simulink model "AFDNFSmodelMPA"  (Simulink 8.8)
settings: Solver=ode45  StartTime=0.0  StopTime=100  FixedStep=1e-3  RelTol=1e-6  EnableMultiTasking=on
InitFcn:
  | run('Methods/AFDSimInit')
  | load('SampleDatcomData.mat')
values from neighbouring files (symbols this model uses):
  nfs = TransferFunction('Plot','true')    [Main.m]    (also in NFSDatabase.sldd = SI
                Imperial
                28184.4409185639)
undefined symbols (not defined in the file or in its folder): datcom, desired, K_lat, K_long, Kobsvlat, Kobsvlong, lat, latsys, long, longsys, Newton, Raphson, sigbuilder_block
libraries: aerolibutil x13, aerolibtransform2 x1, aerolibasang x1
(part 2 of 3)

== system AFDNFSmodelMPA/Nonlinear Flight Simulator/Forces&Moments/Aero Attributes/Velocity Magnitude ==
  Velocity : Inport
  Dot Product : DotProduct  InputSameDT=on  OutDataTypeStr=Inherit: Inherit via internal rule
  Sqrt : Sqrt  SaturateOnIntegerOverflow=on
  Velocity Magnitude : Outport
  wires:
  Sqrt/1 -> Velocity Magnitude/1  "abs(V)"
  Velocity/1 -> Dot Product/2, Dot Product/1
  Dot Product/1 -> Sqrt/1

== system AFDNFSmodelMPA/Nonlinear Flight Simulator/Forces&Moments/Digital DATCOM v1.0.2/Deflection ==
  CP : Inport
  bus : Inport  Port=2
  "V " : Inport  Port=3
  qbar : Inport  Port=4
  CG : Inport  Port=5
  S ref : Inport  Port=6  Unit=m^2
  b ref : Inport  Port=7  Unit=m  PortDimensions=1
  c bar : Inport  Port=8  Unit=m  PortDimensions=1
  Aerodynamic Forces and Moments : Subsystem
  Delta Coefficients : Subsystem
  delta_Faero : Outport
  delta_Maero : Outport  Port=2
  wires:
  Aerodynamic Forces and Moments/1(Forces) -> delta_Faero/1
  Aerodynamic Forces and Moments/2(Moments) -> delta_Maero/1
  S ref/1 -> Aerodynamic Forces and Moments/6(S ref)
  b ref/1 -> Aerodynamic Forces and Moments/7(b ref)
  qbar/1 -> Aerodynamic Forces and Moments/2(qbar)
  c bar/1 -> Aerodynamic Forces and Moments/8(cbar)
  CG/1 -> Aerodynamic Forces and Moments/3(CG)
  "V "/1 -> Aerodynamic Forces and Moments/5(Vb)
  CP/1 -> Aerodynamic Forces and Moments/4(CP)
  Delta Coefficients/1(delCoeff) -> Aerodynamic Forces and Moments/1(Coefficients)
  bus/1 -> Delta Coefficients/1(bus)

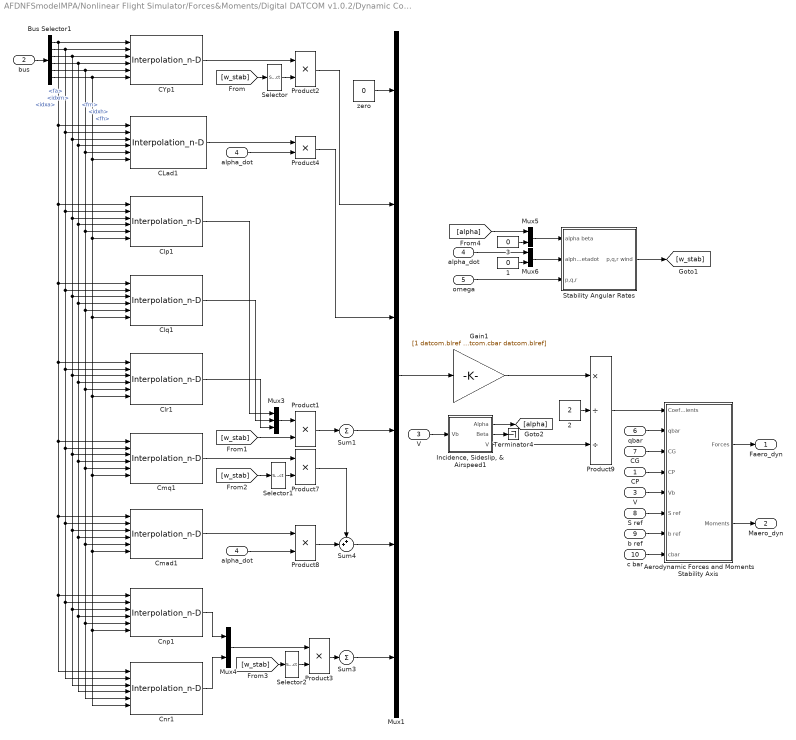
== system AFDNFSmodelMPA/Nonlinear Flight Simulator/Forces&Moments/Digital DATCOM v1.0.2/Dynamic Contribution ==
  CP : Inport
  bus : Inport  Port=2
  V : Inport  Port=3
  alpha_dot : Inport  Port=4  Unit=rad/s
  omega : Inport  Port=5  Unit=rad/s
  qbar : Inport  Port=6
  CG : Inport  Port=7
  S ref : Inport  Port=8  Unit=m^2
  b ref : Inport  Port=9  Unit=m  PortDimensions=1
  c bar : Inport  Port=10  Unit=m  PortDimensions=1
  " V " : InportShadow  Port=3
  " alpha_dot " : InportShadow  Port=4  Unit=rad/s
  1 : Constant  Value=0
  2 : Constant  Value=2
  3 : Constant  Value=0
  Aerodynamic Forces and Moments Stability Axis : Subsystem
  Bus Selector1 : BusSelector  OutputSignals=idxa,fa,idxm,fm,idxh,fh
  CLad1 : Interpolation_n-D  NumberOfTableDimensions=3  Table="permute(datcom.clad,[1  2  3])"  OutDataTypeStr=double
      settings: InputPortMap=u0,u1,u2,u3,u4,u5
  CYp1 : Interpolation_n-D  NumberOfTableDimensions=3  Table="permute(datcom.cyp,[1  2  3])"  OutDataTypeStr=double
      settings: InputPortMap=u0,u1,u2,u3,u4,u5
  Clp1 : Interpolation_n-D  NumberOfTableDimensions=3  Table="permute(datcom.clp,[1  2  3])"  OutDataTypeStr=double
      settings: InputPortMap=u0,u1,u2,u3,u4,u5
  Clq1 : Interpolation_n-D  NumberOfTableDimensions=3  Table="permute(datcom.clq,[1  2  3])"  OutDataTypeStr=double
      settings: InputPortMap=u0,u1,u2,u3,u4,u5
  Clr1 : Interpolation_n-D  NumberOfTableDimensions=3  Table="permute(datcom.clr,[1  2  3])"  OutDataTypeStr=double
      settings: InputPortMap=u0,u1,u2,u3,u4,u5
  Cmad1 : Interpolation_n-D  NumberOfTableDimensions=3  Table="permute(datcom.cmad,[1  2  3])"  OutDataTypeStr=double
      settings: InputPortMap=u0,u1,u2,u3,u4,u5
  Cmq1 : Interpolation_n-D  NumberOfTableDimensions=3  Table="permute(datcom.cmq,[1  2  3])"  OutDataTypeStr=double
      settings: InputPortMap=u0,u1,u2,u3,u4,u5
  Cnp1 : Interpolation_n-D  NumberOfTableDimensions=3  Table="permute(datcom.cnp,[1  2  3])"  OutDataTypeStr=double
      settings: InputPortMap=u0,u1,u2,u3,u4,u5
  Cnr1 : Interpolation_n-D  NumberOfTableDimensions=3  Table="permute(datcom.cnr,[1  2  3])"  OutDataTypeStr=double
      settings: InputPortMap=u0,u1,u2,u3,u4,u5
  Gain1 : Gain  Gain=[1 datcom.blref datcom.cbar datcom.blref datcom.cbar datcom.blref]
  "Incidence, Sideslip, & Airspeed1" : Subsystem
      mask Display:
      | port_label('input',1,'V_b','texmode','on');
      | port_label('output',1,'\alpha','texmode','on');
      | port_label('output',2,'\beta','texmode','on');
      | port_label('output',3,'V','texmode','on');
  Mux1 : Mux  Inputs=6
  Mux3 : Mux  Inputs=3
  Mux4 : Mux  Inputs=2
  Mux5 : Mux  Inputs=2
  Mux6 : Mux  Inputs=2
  Product{1..4,7..8} (6 alike) : Product  RndMeth=Zero
  Product9 : Product  Inputs=*//  RndMeth=Zero
  Selector : Selector  InputPortWidth=3  IndexOptions=Index vector (dialog)  Indices=1  OutputSizes=1
  Selector1 : Selector  InputPortWidth=3  IndexOptions=Index vector (dialog)  Indices=2  OutputSizes=1
  Selector2 : Selector  InputPortWidth=3  IndexOptions=Index vector (dialog)  Indices=[1 3]  OutputSizes=1
  Stability Angular Rates : Subsystem
      mask Display:
      | port_label('input',1,'\alpha \beta','texmode','on');
      | port_label('input',2,'d\alpha/dt d\beta/dt','texmode','on');
      | port_label('input',3,'\omega','texmode','on');
      | port_label('output',1,'\omega_w','texmode','on');
  Sum1 : Sum  Inputs=+
  Sum3 : Sum  Inputs=+
  Sum4 : Sum  Inputs=++|
  Terminator4 : Terminator
  "alpha_dot " : InportShadow  Port=4  Unit=rad/s
  zero : Constant  Value=0
  Faero_dyn : Outport
  Maero_dyn : Outport  Port=2
  wires:
  c bar/1 -> Aerodynamic Forces and Moments Stability Axis/8(cbar)
  b ref/1 -> Aerodynamic Forces and Moments Stability Axis/7(b ref)
  S ref/1 -> Aerodynamic Forces and Moments Stability Axis/6(S ref)
  CLad1/1 -> Product4/1
  Bus Selector1/6 -> Clp1/6, Clq1/6, Clr1/6, Cmq1/6, Cmad1/6, Cnp1/6, Cnr1/6, CLad1/6, CYp1/6  "<fh>"
  Bus Selector1/5 -> Clp1/5, Clq1/5, Clr1/5, Cmq1/5, Cmad1/5, Cnp1/5, Cnr1/5, CLad1/5, CYp1/5  "<idxh>"
  Bus Selector1/4 -> Clp1/4, Clq1/4, Clr1/4, Cmq1/4, Cmad1/4, Cnp1/4, Cnr1/4, CLad1/4, CYp1/4  "<fm>"
  Bus Selector1/3 -> Clp1/3, Clq1/3, Clr1/3, Cmq1/3, Cmad1/3, Cnp1/3, Cnr1/3, CLad1/3, CYp1/3  "<idxm>"
  Bus Selector1/2 -> Clp1/2, Clq1/2, Clr1/2, Cmq1/2, Cmad1/2, Cnp1/2, Cnr1/2, CLad1/2, CYp1/2  "<fa>"
  Bus Selector1/1 -> Clp1/1, Clq1/1, Clr1/1, Cmq1/1, Cmad1/1, Cnp1/1, Cnr1/1, CLad1/1, CYp1/1  "<idxa>"
  bus/1 -> Bus Selector1/1
  " alpha_dot "/1 -> Mux6/1
  omega/1 -> Stability Angular Rates/3(p,q,r)
  Stability Angular Rates/1(p,q,r wind) -> [w_stab]
  Mux1/1 -> Gain1/1
  Cnp1/1 -> Mux4/1
  Cmq1/1 -> Product7/1
  Sum1/1 -> Mux1/4
  Product2/1 -> Mux1/2
  Clq1/1 -> Mux3/2
  Selector/1 -> Product2/2
  CYp1/1 -> Product2/1
  "alpha_dot "/1 -> Product4/2
  [w_stab] -> Selector/1
  Clr1/1 -> Mux3/3
  Clp1/1 -> Mux3/1
  Mux3/1 -> Product1/1
  [w_stab] -> Product1/2
  Product1/1 -> Sum1/1
  [w_stab] -> Selector1/1
  Selector1/1 -> Product7/2
  Product7/1 -> Sum4/1
  Cmad1/1 -> Product8/1
  Product8/1 -> Sum4/2
  alpha_dot/1 -> Product8/2
  Cnr1/1 -> Mux4/2
  [w_stab] -> Selector2/1
  Mux4/1 -> Product3/1
  Selector2/1 -> Product3/2
  Sum3/1 -> Mux1/6
  Product3/1 -> Sum3/1
  Gain1/1 -> Product9/1
  Product9/1 -> Aerodynamic Forces and Moments Stability Axis/1(Coefficients)
  2/1 -> Product9/2
  V/1 -> "Incidence, Sideslip, & Airspeed1"/1(Vb)
  Sum4/1 -> Mux1/5
  Product4/1 -> Mux1/3
  zero/1 -> Mux1/1
  "Incidence, Sideslip, & Airspeed1"/3(V) -> Product9/3
  "Incidence, Sideslip, & Airspeed1"/2(Beta) -> Terminator4/1
  "Incidence, Sideslip, & Airspeed1"/1(Alpha) -> [alpha]
  Aerodynamic Forces and Moments Stability Axis/1(Forces) -> Faero_dyn/1
  qbar/1 -> Aerodynamic Forces and Moments Stability Axis/2(qbar)
  Aerodynamic Forces and Moments Stability Axis/2(Moments) -> Maero_dyn/1
  " V "/1 -> Aerodynamic Forces and Moments Stability Axis/5(Vb)
  3/1 -> Mux5/2
  [alpha] -> Mux5/1
  Mux5/1 -> Stability Angular Rates/1(alpha beta)
  Mux6/1 -> Stability Angular Rates/2(alphadot betadot)
  1/1 -> Mux6/2
  CG/1 -> Aerodynamic Forces and Moments Stability Axis/3(CG)
  CP/1 -> Aerodynamic Forces and Moments Stability Axis/4(CP)

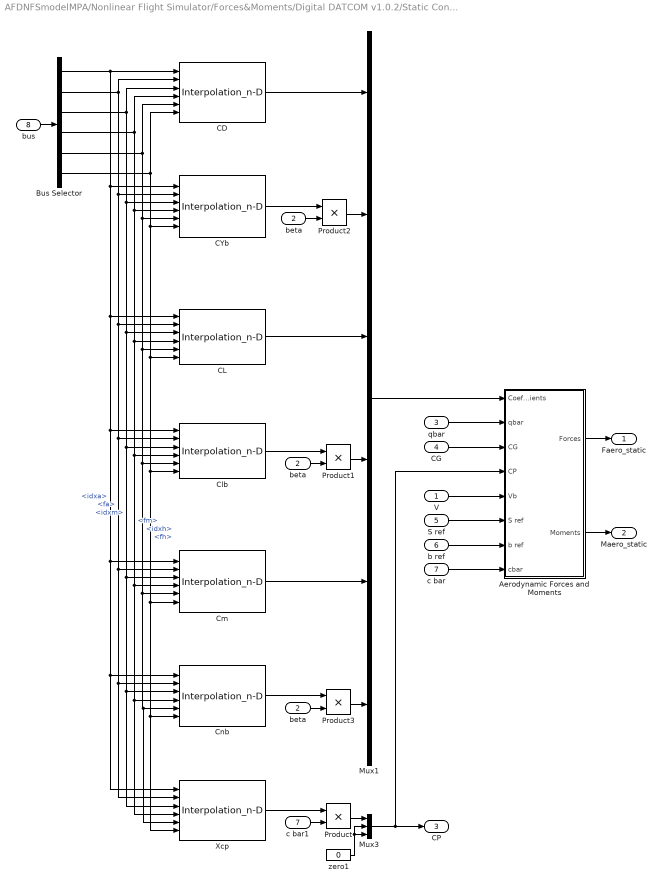
== system AFDNFSmodelMPA/Nonlinear Flight Simulator/Forces&Moments/Digital DATCOM v1.0.2/Static Contribution ==
  "V " : Inport
  beta : Inport  Port=2
  qbar : Inport  Port=3
  CG : Inport  Port=4
  S ref : Inport  Port=5  Unit=m^2
  b ref : Inport  Port=6  Unit=m  PortDimensions=1
  c bar : Inport  Port=7  Unit=m  PortDimensions=1
  bus : Inport  Port=8
  " beta " : InportShadow  Port=2
  Aerodynamic Forces and Moments : Subsystem
  Bus Selector : BusSelector  OutputSignals=idxa,fa,idxm,fm,idxh,fh
  CD : Interpolation_n-D  NumberOfTableDimensions=3  Table=permute(datcom.cd,[1 2 3])  InterpMethod=Flat  ExtrapMethod=Clip  OutDataTypeStr=double
      settings: InputPortMap=u0,u1,u2,u3,u4,u5
  CL : Interpolation_n-D  NumberOfTableDimensions=3  Table=permute(datcom.cl,[1 2 3])  InterpMethod=Flat  ExtrapMethod=Clip  OutDataTypeStr=double
      settings: InputPortMap=u0,u1,u2,u3,u4,u5
  CYb : Interpolation_n-D  NumberOfTableDimensions=3  Table=permute(datcom.cyb,[1 2 3])  InterpMethod=Flat  ExtrapMethod=Clip  OutDataTypeStr=double
      settings: InputPortMap=u0,u1,u2,u3,u4,u5
  Clb : Interpolation_n-D  NumberOfTableDimensions=3  Table=permute(datcom.clb,[1 2 3])  InterpMethod=Flat  ExtrapMethod=Clip  OutDataTypeStr=double
      settings: InputPortMap=u0,u1,u2,u3,u4,u5
  Cm : Interpolation_n-D  NumberOfTableDimensions=3  Table=permute(datcom.cm,[1 2 3])  InterpMethod=Flat  ExtrapMethod=Clip  OutDataTypeStr=double
      settings: InputPortMap=u0,u1,u2,u3,u4,u5
  Cnb : Interpolation_n-D  NumberOfTableDimensions=3  Table=permute(datcom.cnb,[1 2 3])  InterpMethod=Flat  ExtrapMethod=Clip  OutDataTypeStr=double
      settings: InputPortMap=u0,u1,u2,u3,u4,u5
  Mux1 : Mux  Inputs=6
  Mux3 : Mux  Inputs=3
  Product : Product
  Product1 : Product  RndMeth=Zero
  Product2 : Product  RndMeth=Zero
  Product3 : Product  RndMeth=Zero
  Xcp : Interpolation_n-D  NumberOfTableDimensions=3  Table="permute(datcom.xcp,[1  2  3])"  OutDataTypeStr=double
      settings: InputPortMap=u0,u1,u2,u3,u4,u5
  "beta " : InportShadow  Port=2
  c bar1 : InportShadow  Port=7  Unit=m  PortDimensions=1
  zero1 : Constant  Value=0
  Faero_static : Outport
  Maero_static : Outport  Port=2
  "CP " : Outport  Port=3
  wires:
  c bar1/1 -> Product/2
  Product/1 -> Mux3/1
  zero1/1 -> Mux3/3, Mux3/2
  Xcp/1 -> Product/1
  c bar/1 -> Aerodynamic Forces and Moments/8(cbar)
  b ref/1 -> Aerodynamic Forces and Moments/7(b ref)
  S ref/1 -> Aerodynamic Forces and Moments/6(S ref)
  Mux3/1 -> Aerodynamic Forces and Moments/4(CP), "CP "/1
  CG/1 -> Aerodynamic Forces and Moments/3(CG)
  bus/1 -> Bus Selector/1
  Bus Selector/1 -> CD/1, CYb/1, Clb/1, Cnb/1, Xcp/1, Cm/1, CL/1  "<idxa>"
  Bus Selector/2 -> Cnb/2, Xcp/2, Cm/2, Clb/2, CL/2, CYb/2, CD/2  "<fa>"
  Bus Selector/3 -> Cnb/3, Xcp/3, Cm/3, Clb/3, CL/3, CYb/3, CD/3  "<idxm>"
  Bus Selector/4 -> Cnb/4, Xcp/4, Cm/4, Clb/4, CL/4, CYb/4, CD/4  "<fm>"
  Bus Selector/5 -> Cnb/5, Xcp/5, Cm/5, Clb/5, CL/5, CYb/5, CD/5  "<idxh>"
  Bus Selector/6 -> Cnb/6, Xcp/6, Cm/6, Clb/6, CL/6, CYb/6, CD/6  "<fh>"
  CD/1 -> Mux1/1
  CL/1 -> Mux1/3
  CYb/1 -> Product2/1
  beta/1 -> Product2/2
  Clb/1 -> Product1/1
  "beta "/1 -> Product1/2
  Product2/1 -> Mux1/2
  Product1/1 -> Mux1/4
  Cm/1 -> Mux1/5
  Cnb/1 -> Product3/1
  " beta "/1 -> Product3/2
  Product3/1 -> Mux1/6
  Mux1/1 -> Aerodynamic Forces and Moments/1(Coefficients)
  Aerodynamic Forces and Moments/1(Forces) -> Faero_static/1
  qbar/1 -> Aerodynamic Forces and Moments/2(qbar)
  Aerodynamic Forces and Moments/2(Moments) -> Maero_static/1
  "V "/1 -> Aerodynamic Forces and Moments/5(Vb)

== system AFDNFSmodelMPA/Nonlinear Flight Simulator/Forces&Moments/Thrust/Signal Builder ==
  Demux : Demux  Tag=STV Demux  Outputs=1
  FromWs : FromWorkspace  Tag=STV FromWs  VariableName=tuvar  SampleTime=0  SigBuilderData=DataTag1  VnvData=DataTag2
      SigBuilderData=|
      | common.afterFinalStr = 'Extrapolate'
      | common.sampleTime = 0
      | dataSet.timeRange = [0 1200]
      | dataSet.name = 'Thrust Deviation'
      | sbobj.Groups.Name = 'Thrust Deviation'
      | sbobj.Groups.Signals.Name = 'ThrustDeviation'
      | sbobj.Groups.Signals.XData = [0 10 10 12 12 1200]
      | sbobj.Groups.Signals.YData = [1 1 1.05 1.05 1 1]
      | sbobj.Groups.TimeRange = [0 1200]
  ThrustDeviation : Outport  Tag=STV Outport
  wires:
  Demux/1 -> ThrustDeviation/1
  FromWs/1 -> Demux/1

== system AFDNFSmodelMPA/OnBoardComputer/Control System/Trim/Doublet Generated Signal ==
  Constant : Constant  Value=[0;0;0]
  Constant2 : Constant  Value=nfs.trim.delta_e
  Doublet : Subsystem  mask{T_start=10, amp=deg2rad(2), span=1, sampletime=0}
      mask prompts: T_start "Doublet Time"; amp "Amplitude"; span "Time Span"; sampletime "Sample Time"
      mask Display: plot([0,1,1,2,2,3,3,4],[0,0,1,1,-1,-1,0,0])
  Mux : Mux  Inputs=2
  Sum : Sum  Inputs=|++
  Doublet Out : Outport
  wires:
  Sum/1 -> Mux/1
  Constant/1 -> Mux/2
  Doublet/1(Out1) -> Sum/1
  Constant2/1 -> Sum/2
  Mux/1 -> Doublet Out/1

== system AFDNFSmodelMPA/OnBoardComputer/Control System/Trim/Triangular signal span 10 sec ==
  Bus Creator : BusCreator  Inputs=4
  Constant1 : Constant  Value=0
  Constant2 : Constant  Value=nfs.trim.delta_e
  Constant3 : Constant  Value=0
  Constant4 : Constant  Value=0
  Gain{,1..3} (4 alike) : Gain  Gain=pi/180
  Gain4 : Gain  Gain=0
  Gain5 : Gain  Gain=0
  Gain6 : Gain  Gain=0
  Gain7 : Gain
  Signal Builder1 : Subsystem  Tag=STV Subsys  LoadFcn=sigbuilder_block('load');  StartFcn=sigbuilder_block('start');  StopFcn=sigbuilder_block('stop');  ClipboardFcn=sigbuilder_block('clipboard');  mask(Sigbuilder block){tuvar=[0:10]}
      mask help: Simulink:masks:SigbuilderBlock_MD
      mask init:
      | if ~strcmp(get_param(bdroot(gcbh),'SimulationStatus'),'stopped') tuvar = sigbuilder_block('maskInit'); end
      settings: CopyFcn=sigbuilder_block('copy');  DeleteFcn=sigbuilder_block('delete');  ModelCloseFcn=sigbuilder_block('modelClose');  PreSaveFcn=sigbuilder_block('preSave');  PauseFcn=sigbuilder_block('pause');  ContinueFcn=sigbuilder_block('continue');  NameChangeFcn=sigbuilder_block('namechange');  OpenFcn=sigbuilder_block('open',[437.4 199.2 550.2 400.2 ]);  CloseFcn=sigbuilder_block('close');
      mask Display: plot(0, 0, 100, 100,[2, 2, 32, 32, 2], [68, 8, 8, 68, 68],[32, 2], [38, 38], [32, 19, 2],[53, 60, 44], [32, 17, 17, 2],[16, 16, 31, 31]);txt = getActiveGroup(gcbh);text(2, 100, txt,'verticalAlignment', 'top');
  Signal Builder2 : Subsystem  Tag=STV Subsys  LoadFcn=sigbuilder_block('load');  StartFcn=sigbuilder_block('start');  StopFcn=sigbuilder_block('stop');  ClipboardFcn=sigbuilder_block('clipboard');  mask(Sigbuilder block){tuvar=[0:10]}
      mask help: Simulink:masks:SigbuilderBlock_MD
      mask init:
      | if ~strcmp(get_param(bdroot(gcbh),'SimulationStatus'),'stopped') tuvar = sigbuilder_block('maskInit'); end
      settings: CopyFcn=sigbuilder_block('copy');  DeleteFcn=sigbuilder_block('delete');  ModelCloseFcn=sigbuilder_block('modelClose');  PreSaveFcn=sigbuilder_block('preSave');  PauseFcn=sigbuilder_block('pause');  ContinueFcn=sigbuilder_block('continue');  NameChangeFcn=sigbuilder_block('namechange');  OpenFcn=sigbuilder_block('open',[437.25 199.5 550.5 399.75 ]);  CloseFcn=sigbuilder_block('close');
      mask Display: plot(0, 0, 100, 100,[2, 2, 32, 32, 2], [68, 8, 8, 68, 68],[32, 2], [38, 38], [32, 19, 2],[53, 60, 44], [32, 17, 17, 2],[16, 16, 31, 31]);txt = getActiveGroup(gcbh);text(2, 100, txt,'verticalAlignment', 'top');
  Signal Builder3 : Subsystem  Tag=STV Subsys  LoadFcn=sigbuilder_block('load');  StartFcn=sigbuilder_block('start');  StopFcn=sigbuilder_block('stop');  ClipboardFcn=sigbuilder_block('clipboard');  mask(Sigbuilder block){tuvar=[0:10]}
      mask help: Simulink:masks:SigbuilderBlock_MD
      mask init:
      | if ~strcmp(get_param(bdroot(gcbh),'SimulationStatus'),'stopped') tuvar = sigbuilder_block('maskInit'); end
      settings: CopyFcn=sigbuilder_block('copy');  DeleteFcn=sigbuilder_block('delete');  ModelCloseFcn=sigbuilder_block('modelClose');  PreSaveFcn=sigbuilder_block('preSave');  PauseFcn=sigbuilder_block('pause');  ContinueFcn=sigbuilder_block('continue');  NameChangeFcn=sigbuilder_block('namechange');  OpenFcn=sigbuilder_block('open',[437.25 199.5 550.5 399.75 ]);  CloseFcn=sigbuilder_block('close');
      mask Display: plot(0, 0, 100, 100,[2, 2, 32, 32, 2], [68, 8, 8, 68, 68],[32, 2], [38, 38], [32, 19, 2],[53, 60, 44], [32, 17, 17, 2],[16, 16, 31, 31]);txt = getActiveGroup(gcbh);text(2, 100, txt,'verticalAlignment', 'top');
  Signal Builder4 : Subsystem  Tag=STV Subsys  LoadFcn=sigbuilder_block('load');  StartFcn=sigbuilder_block('start');  StopFcn=sigbuilder_block('stop');  ClipboardFcn=sigbuilder_block('clipboard');  mask(Sigbuilder block){tuvar=[0:10]}
      mask help: Simulink:masks:SigbuilderBlock_MD
      mask init:
      | if ~strcmp(get_param(bdroot(gcbh),'SimulationStatus'),'stopped') tuvar = sigbuilder_block('maskInit'); end
      settings: CopyFcn=sigbuilder_block('copy');  DeleteFcn=sigbuilder_block('delete');  ModelCloseFcn=sigbuilder_block('modelClose');  PreSaveFcn=sigbuilder_block('preSave');  PauseFcn=sigbuilder_block('pause');  ContinueFcn=sigbuilder_block('continue');  NameChangeFcn=sigbuilder_block('namechange');  OpenFcn=sigbuilder_block('open',[437.25 199.5 550.5 399.75 ]);  CloseFcn=sigbuilder_block('close');
      mask Display: plot(0, 0, 100, 100,[2, 2, 32, 32, 2], [68, 8, 8, 68, 68],[32, 2], [38, 38], [32, 19, 2],[53, 60, 44], [32, 17, 17, 2],[16, 16, 31, 31]);txt = getActiveGroup(gcbh);text(2, 100, txt,'verticalAlignment', 'top');
  Sum{,1..3} (4 alike) : Sum  Inputs=++|
  Tri : Outport
  wires:
  Signal Builder1/1(Normalized Elevator(deg)) -> Gain/1
  Constant2/1 -> Sum/1
  Gain/1 -> Sum/2
  Signal Builder2/1(Normalized Flap(deg)) -> Gain1/1
  Constant1/1 -> Sum1/1
  Gain1/1 -> Sum1/2
  Signal Builder3/1(Normalized Alileron(deg)) -> Gain2/1
  Constant3/1 -> Sum2/1
  Gain2/1 -> Sum2/2
  Signal Builder4/1(Normalized Rudder(deg)) -> Gain3/1
  Constant4/1 -> Sum3/1
  Gain3/1 -> Sum3/2
  Sum/1 -> Gain7/1
  Sum1/1 -> Gain6/1
  Sum2/1 -> Gain5/1
  Sum3/1 -> Gain4/1
  Gain6/1 -> Bus Creator/2  "delta_f"
  Gain5/1 -> Bus Creator/3  "delta_a"
  Gain7/1 -> Bus Creator/1  "delta_e"
  Gain4/1 -> Bus Creator/4  "delta_r"
  Bus Creator/1 -> Tri/1

== system AFDNFSmodelMPA/Nonlinear Flight Simulator/6DoF Nonlinear Flight Equations of Motion (Rigid Body)/AngularAcceleration(Omegadot)/Cross Product/Subsystem2 ==
  A : Inport
  B : Inport  Port=2
  Demux : Demux  Outputs=3
  Demux1 : Demux  Outputs=3
  Mux : Mux  Inputs=3
  i x j : Product  SaturateOnIntegerOverflow=on  InputSameDT=on  OutDataTypeStr=Inherit: Same as first input
  j x k : Product  SaturateOnIntegerOverflow=on  InputSameDT=on  OutDataTypeStr=Inherit: Same as first input
  k x i : Product  SaturateOnIntegerOverflow=on  InputSameDT=on  OutDataTypeStr=Inherit: Same as first input
  Out1 : Outport
  wires:
  Demux1/3 -> j x k/2
  Demux/2 -> j x k/1
  Demux/3 -> k x i/1
  Demux1/1 -> k x i/2
  Demux1/2 -> i x j/2
  Demux/1 -> i x j/1
  i x j/1 -> Mux/3
  k x i/1 -> Mux/2
  j x k/1 -> Mux/1
  B/1 -> Demux1/1
  A/1 -> Demux/1
  Mux/1 -> Out1/1

== system AFDNFSmodelMPA/Nonlinear Flight Simulator/6DoF Nonlinear Flight Equations of Motion (Rigid Body)/AngularAcceleration(Omegadot)/Cross Product/Subsystem3 ==
  A : Inport
  B : Inport  Port=2
  Demux : Demux  Outputs=3
  Demux1 : Demux  Outputs=3
  Mux : Mux  Inputs=3
  i x k : Product  SaturateOnIntegerOverflow=on  InputSameDT=on  OutDataTypeStr=Inherit: Same as first input
  j x i : Product  SaturateOnIntegerOverflow=on  InputSameDT=on  OutDataTypeStr=Inherit: Same as first input
  k x j : Product  SaturateOnIntegerOverflow=on  InputSameDT=on  OutDataTypeStr=Inherit: Same as first input
  Out2 : Outport
  wires:
  j x i/1 -> Mux/3
  i x k/1 -> Mux/2
  k x j/1 -> Mux/1
  Mux/1 -> Out2/1
  Demux1/1 -> j x i/2
  Demux/2 -> j x i/1
  Demux1/3 -> i x k/2
  Demux/1 -> i x k/1
  Demux1/2 -> k x j/2
  Demux/3 -> k x j/1
  B/1 -> Demux1/1
  A/1 -> Demux/1

== system AFDNFSmodelMPA/Nonlinear Flight Simulator/6DoF Nonlinear Flight Equations of Motion (Rigid Body)/Linear Acceleration(Vdot)/Cross Product/Subsystem2 ==
  A : Inport
  B : Inport  Port=2
  Demux : Demux  Outputs=3
  Demux1 : Demux  Outputs=3
  Mux : Mux  Inputs=3
  i x j : Product  SaturateOnIntegerOverflow=on  InputSameDT=on  OutDataTypeStr=Inherit: Same as first input
  j x k : Product  SaturateOnIntegerOverflow=on  InputSameDT=on  OutDataTypeStr=Inherit: Same as first input
  k x i : Product  SaturateOnIntegerOverflow=on  InputSameDT=on  OutDataTypeStr=Inherit: Same as first input
  Out1 : Outport
  wires:
  Demux1/3 -> j x k/2
  Demux/2 -> j x k/1
  Demux/3 -> k x i/1
  Demux1/1 -> k x i/2
  Demux1/2 -> i x j/2
  Demux/1 -> i x j/1
  i x j/1 -> Mux/3
  k x i/1 -> Mux/2
  j x k/1 -> Mux/1
  B/1 -> Demux1/1
  A/1 -> Demux/1
  Mux/1 -> Out1/1

== system AFDNFSmodelMPA/Nonlinear Flight Simulator/6DoF Nonlinear Flight Equations of Motion (Rigid Body)/Linear Acceleration(Vdot)/Cross Product/Subsystem3 ==
  A : Inport
  B : Inport  Port=2
  Demux : Demux  Outputs=3
  Demux1 : Demux  Outputs=3
  Mux : Mux  Inputs=3
  i x k : Product  SaturateOnIntegerOverflow=on  InputSameDT=on  OutDataTypeStr=Inherit: Same as first input
  j x i : Product  SaturateOnIntegerOverflow=on  InputSameDT=on  OutDataTypeStr=Inherit: Same as first input
  k x j : Product  SaturateOnIntegerOverflow=on  InputSameDT=on  OutDataTypeStr=Inherit: Same as first input
  Out2 : Outport
  wires:
  j x i/1 -> Mux/3
  i x k/1 -> Mux/2
  k x j/1 -> Mux/1
  Mux/1 -> Out2/1
  Demux1/1 -> j x i/2
  Demux/2 -> j x i/1
  Demux1/3 -> i x k/2
  Demux/1 -> i x k/1
  Demux1/2 -> k x j/2
  Demux/3 -> k x j/1
  B/1 -> Demux1/1
  A/1 -> Demux/1

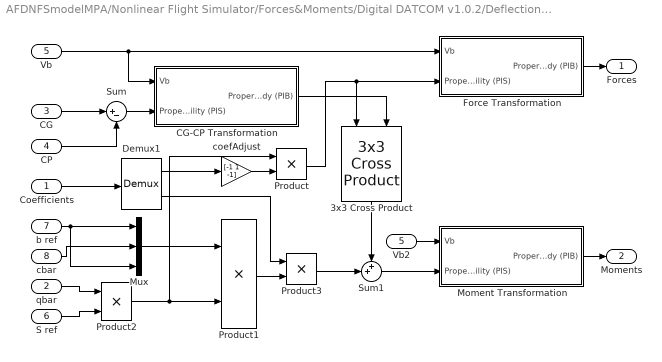
== system AFDNFSmodelMPA/Nonlinear Flight Simulator/Forces&Moments/Digital DATCOM v1.0.2/Deflection/Aerodynamic Forces and Moments ==
  Coefficients : Inport
  qbar : Inport  Port=2  Unit=Pa
  CG : Inport  Port=3  Unit=m  PortDimensions=[3, 1]
  CP : Inport  Port=4  Unit=m  PortDimensions=[3,1]
  Vb : Inport  Port=5
  S ref : Inport  Port=6  Unit=m^2  PortDimensions=1
  b ref : Inport  Port=7  Unit=m  PortDimensions=1
  cbar : Inport  Port=8  Unit=m  PortDimensions=1
  3x3 Cross Product : aerolibutil/3x3 Cross Product
  CG-CP Transformation : Subsystem
  Demux1 : Demux  Outputs=[3,3]
  Force Transformation : Subsystem
  Moment Transformation : Subsystem
  Mux : Mux  Inputs=3
  Product{,1..3} (4 alike) : Product  SaturateOnIntegerOverflow=on  InputSameDT=on  OutDataTypeStr=Inherit: Same as first input
  Sum : Sum  Inputs=|+-  SaturateOnIntegerOverflow=on
  Sum1 : Sum  Inputs=++|  SaturateOnIntegerOverflow=on  InputSameDT=on  OutDataTypeStr=Inherit: Same as first input
  Vb2 : InportShadow  Port=5
  coefAdjust : Gain  Gain="[-1  1 -1]"
  Forces : Outport  Unit=N
  Moments : Outport  Port=2  Unit=N
  wires:
  Vb2/1 -> Moment Transformation/1(Vb)
  Sum1/1 -> Moment Transformation/2(Property-In-Stability (PIS))
  S ref/1 -> Product2/2
  Mux/1 -> Product1/1
  b ref/1 -> Mux/3, Mux/1
  cbar/1 -> Mux/2
  3x3 Cross Product/1 -> Sum1/1
  Product1/1 -> Product3/2
  Coefficients/1 -> Demux1/1
  Demux1/2 -> Product3/1
  qbar/1 -> Product2/1
  Product2/1 -> Product1/2, Product/1
  Product3/1 -> Sum1/2
  Demux1/1 -> coefAdjust/1
  Product/1 -> Force Transformation/2(Property-In-Stability (PIS)), 3x3 Cross Product/1
  Force Transformation/1(Property-In-Body (PIB)) -> Forces/1
  Moment Transformation/1(Property-In-Body (PIB)) -> Moments/1
  coefAdjust/1 -> Product/2
  CG/1 -> Sum/1
  CP/1 -> Sum/2
  Sum/1 -> CG-CP Transformation/2(Property-In-Stability (PIS))
  CG-CP Transformation/1(Property-In-Body (PIB)) -> 3x3 Cross Product/2
  Vb/1 -> Force Transformation/1(Vb), CG-CP Transformation/1(Vb)

== system AFDNFSmodelMPA/Nonlinear Flight Simulator/Forces&Moments/Digital DATCOM v1.0.2/Deflection/Delta Coefficients ==
  bus : Inport
  Aileron Deflaction : Subsystem
  Elevator Deflaction : Subsystem
  Flap Deflaction : Subsystem
  Sum : Sum  Inputs=+++
  delCoeff : Outport
  wires:
  Sum/1 -> delCoeff/1
  Aileron Deflaction/1(delCoeff_a) -> Sum/3
  Flap Deflaction/1(delCoeff_f) -> Sum/1
  Elevator Deflaction/1(delCoeff_e) -> Sum/2
  bus/1 -> Elevator Deflaction/1(bus), Aileron Deflaction/1(bus), Flap Deflaction/1(bus)

== system AFDNFSmodelMPA/Nonlinear Flight Simulator/Forces&Moments/Digital DATCOM v1.0.2/Dynamic Contribution/Aerodynamic Forces and Moments Stability Axis ==
  Coefficients : Inport
  qbar : Inport  Port=2  Unit=Pa
  CG : Inport  Port=3  Unit=m  PortDimensions=[3, 1]
  CP : Inport  Port=4  Unit=m  PortDimensions=[3,1]
  Vb : Inport  Port=5
  S ref : Inport  Port=6  Unit=m^2  PortDimensions=1
  b ref : Inport  Port=7  Unit=m  PortDimensions=1
  cbar : Inport  Port=8  Unit=m  PortDimensions=1
  3x3 Cross Product : aerolibutil/3x3 Cross Product
  CG-CP Transformation : Subsystem
  Demux1 : Demux  Outputs=[3,3]
  Force Transformation : Subsystem
  Moment Transformation : Subsystem
  Mux : Mux  Inputs=3
  Product{,1..3} (4 alike) : Product  SaturateOnIntegerOverflow=on  InputSameDT=on  OutDataTypeStr=Inherit: Same as first input
  Sum : Sum  Inputs=|+-  SaturateOnIntegerOverflow=on
  Sum1 : Sum  Inputs=++|  SaturateOnIntegerOverflow=on  InputSameDT=on  OutDataTypeStr=Inherit: Same as first input
  Vb2 : InportShadow  Port=5
  coefAdjust : Gain  Gain="[-1  1 -1]"
  Forces : Outport  Unit=N
  Moments : Outport  Port=2  Unit=N*m
  wires:
  Vb2/1 -> Moment Transformation/1(Vb)
  Sum1/1 -> Moment Transformation/2(Property-In-Stability (PIS))
  S ref/1 -> Product2/2
  Mux/1 -> Product1/1
  b ref/1 -> Mux/3, Mux/1
  cbar/1 -> Mux/2
  3x3 Cross Product/1 -> Sum1/1
  Product1/1 -> Product3/2
  Coefficients/1 -> Demux1/1
  Demux1/2 -> Product3/1
  qbar/1 -> Product2/1
  Product2/1 -> Product1/2, Product/1
  Product3/1 -> Sum1/2
  Demux1/1 -> coefAdjust/1
  Product/1 -> Force Transformation/2(Property-In-Stability (PIS)), 3x3 Cross Product/1
  Force Transformation/1(Property-In-Body (PIB)) -> Forces/1
  Moment Transformation/1(Property-In-Body (PIB)) -> Moments/1
  coefAdjust/1 -> Product/2
  CG/1 -> Sum/1
  CP/1 -> Sum/2
  Sum/1 -> CG-CP Transformation/2(Property-In-Stability (PIS))
  CG-CP Transformation/1(Property-In-Body (PIB)) -> 3x3 Cross Product/2
  Vb/1 -> Force Transformation/1(Vb), CG-CP Transformation/1(Vb)

== system AFDNFSmodelMPA/Nonlinear Flight Simulator/Forces&Moments/Digital DATCOM v1.0.2/Dynamic Contribution/Incidence, Sideslip, & Airspeed1 ==
  Vb : Inport  Unit=m/s
  Airspeed : Sqrt  AlgorithmType=Newton-Raphson  SaturateOnIntegerOverflow=on
  Dot Product : DotProduct  InputSameDT=on  OutDataTypeStr=Inherit: Inherit via internal rule
  Incidence : Trigonometry  Operator=atan2
  Product : Product  Inputs=*/  SaturateOnIntegerOverflow=on  OutDataTypeStr=Inherit: Same as first input
  Selector : Selector  InputPortWidth=3  IndexOptions=Index vector (dialog)  Indices=[2]  OutputSizes=1
  Selector1 : Selector  InputPortWidth=3  IndexOptions=Index vector (dialog)  Indices=[3]  OutputSizes=1
  Selector2 : Selector  InputPortWidth=3  IndexOptions=Index vector (dialog)  Indices=[1]  OutputSizes=1
  Sideslip : Trigonometry  Operator=asin
  Alpha : Outport  Unit=rad  InitialOutput=0
  Beta : Outport  Port=2  Unit=rad  InitialOutput=0
  V : Outport  Port=3  Unit=m/s  InitialOutput=0
  wires:
  Selector/1 -> Product/1
  Sideslip/1 -> Beta/1
  Vb/1 -> Dot Product/2, Dot Product/1, Selector/1, Selector2/1, Selector1/1
  Incidence/1 -> Alpha/1
  Airspeed/1 -> V/1, Product/2
  Dot Product/1 -> Airspeed/1
  Selector2/1 -> Incidence/2
  Selector1/1 -> Incidence/1
  Product/1 -> Sideslip/1

== system AFDNFSmodelMPA/Nonlinear Flight Simulator/Forces&Moments/Digital DATCOM v1.0.2/Dynamic Contribution/Stability Angular Rates ==
  alpha beta : Inport  Unit=rad
  alphadot betadot : Inport  Port=2  Unit=rad/s
  p,q,r : Inport  Port=3  Unit=rad/s
  Demux : Demux  Outputs=2
  Direction Cosine Matrix Body to Wind : aerolibtransform2/Direction Cosine Matrix Body to Wind
  Disallow CGS : UnitConfiguration  UnitSystems=DataTag0  UnitSystemsStr=English,SI,SI (extended)  AllowAllUnitSystems=off
  Mux : Mux  Inputs=3
  Product : Product  RndMeth=Zero
  Product1 : Product  Multiplication=Matrix(*)  SaturateOnIntegerOverflow=on  InputSameDT=on  OutDataTypeStr=Inherit: Same as first input
  Product2 : Product  RndMeth=Zero
  SinCos : Trigonometry  Operator=sincos
  Subsystem : aerolibasang/Wind Angular Rates/Subsystem
  Sum : Sum  Inputs=|++
  Unary Minus : UnaryMinus
  Unary Minus1 : UnaryMinus
  p,q,r wind : Outport  Unit=rad/s  InitialOutput=0
  wires:
  alpha beta/1 -> Direction Cosine Matrix Body to Wind/1, Subsystem/1
  Subsystem/1 -> SinCos/1
  SinCos/1 -> Product/2
  SinCos/2 -> Product2/2
  Direction Cosine Matrix Body to Wind/1 -> Product1/1
  Sum/1 -> Product1/2
  Product1/1 -> p,q,r wind/1
  Mux/1 -> Sum/1
  p,q,r/1 -> Sum/2
  alphadot betadot/1 -> Demux/1
  Demux/2 -> Product2/1, Product/1
  Demux/1 -> Unary Minus/1
  Product/1 -> Unary Minus1/1
  Product2/1 -> Mux/3
  Unary Minus1/1 -> Mux/1
  Unary Minus/1 -> Mux/2

== system AFDNFSmodelMPA/Nonlinear Flight Simulator/Forces&Moments/Digital DATCOM v1.0.2/Static Contribution/Aerodynamic Forces and Moments ==
  Coefficients : Inport
  qbar : Inport  Port=2  Unit=Pa
  CG : Inport  Port=3  Unit=m  PortDimensions=[3, 1]
  CP : Inport  Port=4  Unit=m  PortDimensions=[3,1]
  Vb : Inport  Port=5
  S ref : Inport  Port=6  Unit=m^2  PortDimensions=1
  b ref : Inport  Port=7  Unit=m  PortDimensions=1
  cbar : Inport  Port=8  Unit=m  PortDimensions=1
  3x3 Cross Product : aerolibutil/3x3 Cross Product
  CG-CP Transformation : Subsystem
  Demux1 : Demux  Outputs=[3,3]
  Force Transformation : Subsystem
  Moment Transformation : Subsystem
  Mux : Mux  Inputs=3
  Product{,1..3} (4 alike) : Product  SaturateOnIntegerOverflow=on  InputSameDT=on  OutDataTypeStr=Inherit: Same as first input
  Sum : Sum  Inputs=|+-  SaturateOnIntegerOverflow=on
  Sum1 : Sum  Inputs=++|  SaturateOnIntegerOverflow=on  InputSameDT=on  OutDataTypeStr=Inherit: Same as first input
  Vb2 : InportShadow  Port=5
  coefAdjust : Gain  Gain="[-1  1 -1]"
  Forces : Outport  Unit=N
  Moments : Outport  Port=2  Unit=N*m
  wires:
  Vb2/1 -> Moment Transformation/1(Vb)
  Sum1/1 -> Moment Transformation/2(Property-In-Stability (PIS))
  S ref/1 -> Product2/2
  Mux/1 -> Product1/1
  b ref/1 -> Mux/3, Mux/1
  cbar/1 -> Mux/2
  3x3 Cross Product/1 -> Sum1/1
  Product1/1 -> Product3/2
  Coefficients/1 -> Demux1/1
  Demux1/2 -> Product3/1
  qbar/1 -> Product2/1
  Product2/1 -> Product1/2, Product/1
  Product3/1 -> Sum1/2
  Demux1/1 -> coefAdjust/1
  Product/1 -> Force Transformation/2(Property-In-Stability (PIS)), 3x3 Cross Product/1
  Force Transformation/1(Property-In-Body (PIB)) -> Forces/1
  Moment Transformation/1(Property-In-Body (PIB)) -> Moments/1
  coefAdjust/1 -> Product/2
  CG/1 -> Sum/1
  CP/1 -> Sum/2
  Sum/1 -> CG-CP Transformation/2(Property-In-Stability (PIS))
  CG-CP Transformation/1(Property-In-Body (PIB)) -> 3x3 Cross Product/2
  Vb/1 -> Force Transformation/1(Vb), CG-CP Transformation/1(Vb)

== system AFDNFSmodelMPA/OnBoardComputer/Control System/Trim/Doublet Generated Signal/Doublet ==
  Step : Step  Time=T_start  After=amp  SampleTime=sampletime
  Step1 : Step  Time=T_start+span/2  After=amp  SampleTime=sampletime
  Step2 : Step  Time=T_start+span/2  After=-amp  SampleTime=sampletime
  Step3 : Step  Time=T_start+span  After=-amp  SampleTime=sampletime
  Sum : Sum  Inputs=|+-
  Sum1 : Sum  Inputs=|+-
  Sum2 : Sum  Inputs=|++
  Out1 : Outport
  wires:
  Step/1 -> Sum/1
  Step1/1 -> Sum/2
  Step2/1 -> Sum1/1
  Step3/1 -> Sum1/2
  Sum/1 -> Sum2/1
  Sum1/1 -> Sum2/2
  Sum2/1 -> Out1/1

== system AFDNFSmodelMPA/OnBoardComputer/Control System/Trim/Triangular signal span 10 sec/Signal Builder1 ==
  Demux : Demux  Tag=STV Demux  Outputs=1
  FromWs : FromWorkspace  Tag=STV FromWs  VariableName=tuvar  SampleTime=0  SigBuilderData=DataTag3  VnvData=DataTag4
      SigBuilderData=|
      | common.afterFinalStr = 'Extrapolate'
      | common.sampleTime = 0
      | dataSet.timeRange = [10 20]
      | dataSet.name = 'Group 1'
      | sbobj.Groups.Name = 'Group 1'
      | sbobj.Groups.Signals.Name = 'Normalized Elevator(deg)'
      | sbobj.Groups.Signals.XData = [10 11 12 13 14 15 16 17 20]
      | sbobj.Groups.Signals.YData = [0 0 0.25 0 -0.25 0 0 0 0]
      | sbobj.Groups.TimeRange = [10 20]
  Normalized Elevator(deg) : Outport  Tag=STV Outport
  wires:
  FromWs/1 -> Demux/1
  Demux/1 -> Normalized Elevator(deg)/1

== system AFDNFSmodelMPA/OnBoardComputer/Control System/Trim/Triangular signal span 10 sec/Signal Builder2 ==
  Demux : Demux  Tag=STV Demux  Outputs=1
  FromWs : FromWorkspace  Tag=STV FromWs  VariableName=tuvar  SampleTime=0  SigBuilderData=DataTag5  VnvData=DataTag6
      SigBuilderData=|
      | common.afterFinalStr = 'Extrapolate'
      | common.sampleTime = 0
      | dataSet.timeRange = [10 20]
      | dataSet.name = 'Group 1'
      | sbobj.Groups.Name = 'Group 1'
      | sbobj.Groups.Signals.Name = 'Normalized Flap(deg)'
      | sbobj.Groups.Signals.XData = [10 11 12 13 14 15 16 17 20]
      | sbobj.Groups.Signals.YData = [0 0 0 0 0 0 0 0 0]
      | sbobj.Groups.TimeRange = [10 20]
  Normalized Flap(deg) : Outport  Tag=STV Outport
  wires:
  Demux/1 -> Normalized Flap(deg)/1
  FromWs/1 -> Demux/1

== system AFDNFSmodelMPA/OnBoardComputer/Control System/Trim/Triangular signal span 10 sec/Signal Builder3 ==
  Demux : Demux  Tag=STV Demux  Outputs=1
  FromWs : FromWorkspace  Tag=STV FromWs  VariableName=tuvar  SampleTime=0  SigBuilderData=DataTag7  VnvData=DataTag8
      SigBuilderData=|
      | common.afterFinalStr = 'Extrapolate'
      | common.sampleTime = 0
      | dataSet.timeRange = [10 20]
      | dataSet.name = 'Group 1'
      | sbobj.Groups.Name = 'Group 1'
      | sbobj.Groups.Signals.Name = 'Normalized Alileron(deg)'
      | sbobj.Groups.Signals.XData = [10 11 12 13 14 15 16 17 20]
      | sbobj.Groups.Signals.YData = [0 0 0.6 0 -0.6 0 0 0 0]
      | sbobj.Groups.TimeRange = [10 20]
  Normalized Alileron(deg) : Outport  Tag=STV Outport
  wires:
  FromWs/1 -> Demux/1
  Demux/1 -> Normalized Alileron(deg)/1

== system AFDNFSmodelMPA/OnBoardComputer/Control System/Trim/Triangular signal span 10 sec/Signal Builder4 ==
  Demux : Demux  Tag=STV Demux  Outputs=1
  FromWs : FromWorkspace  Tag=STV FromWs  VariableName=tuvar  SampleTime=0  SigBuilderData=DataTag9  VnvData=DataTag10
      SigBuilderData=|
      | common.afterFinalStr = 'Extrapolate'
      | common.sampleTime = 0
      | dataSet.timeRange = [10 20]
      | dataSet.name = 'Group 1'
      | sbobj.Groups.Name = 'Group 1'
      | sbobj.Groups.Signals.Name = 'Normalized Rudder(deg)'
      | sbobj.Groups.Signals.XData = [10 11 12 13 14 15 16 17 20]
      | sbobj.Groups.Signals.YData = [0 0 0.6 0 -0.6 0 0 0 0]
      | sbobj.Groups.TimeRange = [10 20]
  Normalized Rudder(deg) : Outport  Tag=STV Outport
  wires:
  Demux/1 -> Normalized Rudder(deg)/1
  FromWs/1 -> Demux/1

== system AFDNFSmodelMPA/Nonlinear Flight Simulator/Forces&Moments/Digital DATCOM v1.0.2/Deflection/Aerodynamic Forces and Moments/CG-CP Transformation ==
  Vb : Inport
  Property-In-Stability (PIS) : Inport  Port=2
  Body2Stability : Subsystem
  "Incidence, Sideslip, & Airspeed" : Subsystem
      mask Display:
      | port_label('input',1,'V_b','texmode','on');
      | port_label('output',1,'\alpha','texmode','on');
      | port_label('output',2,'\beta','texmode','on');
      | port_label('output',3,'V','texmode','on');
  Product : Product  Multiplication=Matrix(*)  RndMeth=Zero
  Terminator : Terminator
  Terminator1 : Terminator
  Transpose : Math  Operator=transpose  SaturateOnIntegerOverflow=on
  Property-In-Body (PIB) : Outport
  wires:
  Product/1 -> Property-In-Body (PIB)/1
  Property-In-Stability (PIS)/1 -> Product/2
  "Incidence, Sideslip, & Airspeed"/1(Alpha) -> Body2Stability/1(alpha)
  Body2Stability/1(Ts/b) -> Transpose/1
  Transpose/1 -> Product/1  "Stability2Body"
  Vb/1 -> "Incidence, Sideslip, & Airspeed"/1(Vb)
  "Incidence, Sideslip, & Airspeed"/2(Beta) -> Terminator/1
  "Incidence, Sideslip, & Airspeed"/3(V) -> Terminator1/1

== system AFDNFSmodelMPA/Nonlinear Flight Simulator/Forces&Moments/Digital DATCOM v1.0.2/Deflection/Aerodynamic Forces and Moments/Force Transformation ==
  Vb : Inport
  Property-In-Stability (PIS) : Inport  Port=2
  Body2Stability : Subsystem
  "Incidence, Sideslip, & Airspeed" : Subsystem
      mask Display:
      | port_label('input',1,'V_b','texmode','on');
      | port_label('output',1,'\alpha','texmode','on');
      | port_label('output',2,'\beta','texmode','on');
      | port_label('output',3,'V','texmode','on');
  Product : Product  Multiplication=Matrix(*)  RndMeth=Zero
  Terminator : Terminator
  Terminator1 : Terminator
  Transpose : Math  Operator=transpose  SaturateOnIntegerOverflow=on
  Property-In-Body (PIB) : Outport
  wires:
  Product/1 -> Property-In-Body (PIB)/1
  Property-In-Stability (PIS)/1 -> Product/2
  "Incidence, Sideslip, & Airspeed"/1(Alpha) -> Body2Stability/1(alpha)
  Body2Stability/1(Ts/b) -> Transpose/1
  Transpose/1 -> Product/1  "Stability2Body"
  Vb/1 -> "Incidence, Sideslip, & Airspeed"/1(Vb)
  "Incidence, Sideslip, & Airspeed"/2(Beta) -> Terminator/1
  "Incidence, Sideslip, & Airspeed"/3(V) -> Terminator1/1

== system AFDNFSmodelMPA/Nonlinear Flight Simulator/Forces&Moments/Digital DATCOM v1.0.2/Deflection/Aerodynamic Forces and Moments/Moment Transformation ==
  Vb : Inport
  Property-In-Stability (PIS) : Inport  Port=2
  Body2Stability : Subsystem
  "Incidence, Sideslip, & Airspeed" : Subsystem
      mask Display:
      | port_label('input',1,'V_b','texmode','on');
      | port_label('output',1,'\alpha','texmode','on');
      | port_label('output',2,'\beta','texmode','on');
      | port_label('output',3,'V','texmode','on');
  Product : Product  Multiplication=Matrix(*)  RndMeth=Zero
  Terminator : Terminator
  Terminator1 : Terminator
  Transpose : Math  Operator=transpose  SaturateOnIntegerOverflow=on
  Property-In-Body (PIB) : Outport
  wires:
  "Incidence, Sideslip, & Airspeed"/3(V) -> Terminator1/1
  "Incidence, Sideslip, & Airspeed"/2(Beta) -> Terminator/1
  Vb/1 -> "Incidence, Sideslip, & Airspeed"/1(Vb)
  Transpose/1 -> Product/1  "Stability2Body"
  Body2Stability/1(Ts/b) -> Transpose/1
  "Incidence, Sideslip, & Airspeed"/1(Alpha) -> Body2Stability/1(alpha)
  Property-In-Stability (PIS)/1 -> Product/2
  Product/1 -> Property-In-Body (PIB)/1

== system AFDNFSmodelMPA/Nonlinear Flight Simulator/Forces&Moments/Digital DATCOM v1.0.2/Deflection/Delta Coefficients/Aileron Deflaction ==
  bus : Inport
  Bus Selector : BusSelector  OutputSignals=idxa,fa,idxm,fm,idxh,fh,idxd_a,fd_a
  Bus Selector1 : BusSelector  OutputSignals=idxa,fa,idxm,fm,idxh,fh,idxd_a,fd_a
  Constant{1,4..6} (4 alike) : Constant  Value=0
  DCl : Interpolation_n-D  NumberOfTableDimensions=4  Table=permute(datcom.dcl_de,[1 2 3 4])  RemoveProtectionIndex=on
      settings: InputPortMap=u0,u1,u2,u3,u4,u5,u6,u7
  DCn : Interpolation_n-D  NumberOfTableDimensions=4  Table=permute(datcom.dcdi_de,[1 2 3 4])  RemoveProtectionIndex=on
      settings: InputPortMap=u0,u1,u2,u3,u4,u5,u6,u7
  Mux1 : Mux  Inputs=6
  delCoeff_a : Outport
  wires:
  Bus Selector/7 -> DCn/7  "<idxd_a>"
  Bus Selector/3 -> DCn/3  "<idxm>"
  Bus Selector1/7 -> DCl/7  "<idxd_a>"
  Bus Selector1/3 -> DCl/3  "<idxm>"
  DCl/1 -> Mux1/4  "Cl_a"
  DCn/1 -> Mux1/6  "Cn_a"
  Constant6/1 -> Mux1/1  "CD_a"
  Constant1/1 -> Mux1/2  "CY_a"
  Constant5/1 -> Mux1/3  "CL_e"
  Constant4/1 -> Mux1/5  "Cm_a"
  bus/1 -> Bus Selector/1, Bus Selector1/1
  Bus Selector1/4 -> DCl/4  "<fm>"
  Bus Selector1/6 -> DCl/6  "<fh>"
  Bus Selector1/8 -> DCl/8  "<fd_a>"
  Bus Selector1/2 -> DCl/2  "<fa>"
  Bus Selector1/5 -> DCl/5  "<idxh>"
  Bus Selector1/1 -> DCl/1  "<idxa>"
  Mux1/1 -> delCoeff_a/1
  Bus Selector/6 -> DCn/6  "<fh>"
  Bus Selector/8 -> DCn/8  "<fd_a>"
  Bus Selector/1 -> DCn/1  "<idxa>"
  Bus Selector/2 -> DCn/2  "<fa>"
  Bus Selector/5 -> DCn/5  "<idxh>"
  Bus Selector/4 -> DCn/4  "<fm>"

== system AFDNFSmodelMPA/Nonlinear Flight Simulator/Forces&Moments/Digital DATCOM v1.0.2/Deflection/Delta Coefficients/Elevator Deflaction ==
  bus : Inport
  Bus Selector : BusSelector  OutputSignals=idxa,fa,idxm,fm,idxh,fh,idxd_e,fd_e
  Bus Selector1 : BusSelector  OutputSignals=idxa,fa,idxm,fm,idxh,fh,idxd_e,fd_e
  Bus Selector2 : BusSelector  OutputSignals=idxa,fa,idxm,fm,idxh,fh,idxd_e,fd_e
  Constant1 : Constant  Value=0
  Constant2 : Constant  Value=0
  Constant3 : Constant  Value=0
  DCDI : Interpolation_n-D  NumberOfTableDimensions=4  Table=permute(datcom.dcdi_de,[1 2 3 4])  RemoveProtectionIndex=on
      settings: InputPortMap=u0,u1,u2,u3,u4,u5,u6,u7
  DCL : Interpolation_n-D  NumberOfTableDimensions=4  Table=permute(datcom.dcl_de,[1 2 3 4])  RemoveProtectionIndex=on
      settings: InputPortMap=u0,u1,u2,u3,u4,u5,u6,u7
  DCm : Interpolation_n-D  NumberOfTableDimensions=4  Table=permute(datcom.dcm_de,[1 2 3 4])  RemoveProtectionIndex=on
      settings: InputPortMap=u0,u1,u2,u3,u4,u5,u6,u7
  Mux1 : Mux  Inputs=6
  delCoeff_e : Outport
  wires:
  Bus Selector2/3 -> DCm/3  "<idxm>"
  Bus Selector2/7 -> DCm/7  "<idxd_e>"
  Bus Selector1/7 -> DCL/7  "<idxd_e>"
  Bus Selector1/3 -> DCL/3  "<idxm>"
  Bus Selector/3 -> DCDI/3  "<idxm>"
  Bus Selector/7 -> DCDI/7  "<idxd_e>"
  Constant2/1 -> Mux1/4  "Cl_e"
  Constant3/1 -> Mux1/6  "Cn_e"
  DCDI/1 -> Mux1/1  "CD_e"
  Constant1/1 -> Mux1/2  "CY_e"
  DCL/1 -> Mux1/3  "CL_e"
  DCm/1 -> Mux1/5  "Cm_e"
  Bus Selector/4 -> DCDI/4  "<fm>"
  Bus Selector/5 -> DCDI/5  "<idxh>"
  Bus Selector/2 -> DCDI/2  "<fa>"
  Bus Selector/1 -> DCDI/1  "<idxa>"
  Bus Selector/8 -> DCDI/8  "<fd_e>"
  Bus Selector/6 -> DCDI/6  "<fh>"
  Mux1/1 -> delCoeff_e/1
  Bus Selector1/1 -> DCL/1  "<idxa>"
  Bus Selector1/5 -> DCL/5  "<idxh>"
  Bus Selector1/2 -> DCL/2  "<fa>"
  Bus Selector2/1 -> DCm/1  "<idxa>"
  Bus Selector2/8 -> DCm/8  "<fd_e>"
  Bus Selector2/5 -> DCm/5  "<idxh>"
  Bus Selector2/4 -> DCm/4  "<fm>"
  Bus Selector2/2 -> DCm/2  "<fa>"
  Bus Selector2/6 -> DCm/6  "<fh>"
  Bus Selector1/8 -> DCL/8  "<fd_e>"
  Bus Selector1/6 -> DCL/6  "<fh>"
  Bus Selector1/4 -> DCL/4  "<fm>"
  bus/1 -> Bus Selector/1, Bus Selector1/1, Bus Selector2/1

== system AFDNFSmodelMPA/Nonlinear Flight Simulator/Forces&Moments/Digital DATCOM v1.0.2/Deflection/Delta Coefficients/Flap Deflaction ==
  bus : Inport
  Bus Selector : BusSelector  OutputSignals=idxa,fa,idxm,fm,idxh,fh,idxd_f,fd_f
  Bus Selector1 : BusSelector  OutputSignals=idxa,fa,idxm,fm,idxh,fh,idxd_f,fd_f
  Bus Selector4 : BusSelector  OutputSignals=idxa,fa,idxm,fm,idxh,fh,idxd_f,fd_f
  Constant1 : Constant  Value=0
  Constant2 : Constant  Value=0
  Constant3 : Constant  Value=0
  DCDI : Interpolation_n-D  NumberOfTableDimensions=4  Table=permute(datcom.dcdi_df,[1 2 3 4])  RemoveProtectionIndex=on
      settings: InputPortMap=u0,u1,u2,u3,u4,u5,u6,u7
  DCL : Interpolation_n-D  NumberOfTableDimensions=4  Table=permute(datcom.dcl_df,[1 2 3 4])  RemoveProtectionIndex=on
      settings: InputPortMap=u0,u1,u2,u3,u4,u5,u6,u7
  DCm : Interpolation_n-D  NumberOfTableDimensions=4  Table=permute(datcom.dcm_df,[1 2 3 4])  RemoveProtectionIndex=on
      settings: InputPortMap=u0,u1,u2,u3,u4,u5,u6,u7
  Mux1 : Mux  Inputs=6
  delCoeff_f : Outport
  wires:
  Bus Selector4/3 -> DCm/3  "<idxm>"
  Bus Selector4/7 -> DCm/7  "<idxd_f>"
  Bus Selector1/7 -> DCL/7  "<idxd_f>"
  Bus Selector1/3 -> DCL/3  "<idxm>"
  Bus Selector/7 -> DCDI/7  "<idxd_f>"
  Bus Selector/3 -> DCDI/3  "<idxm>"
  Constant2/1 -> Mux1/4  "Cl_f"
  Constant3/1 -> Mux1/6  "Cn_f"
  bus/1 -> Bus Selector1/1, Bus Selector4/1, Bus Selector/1
  Bus Selector1/4 -> DCL/4  "<fm>"
  Bus Selector1/6 -> DCL/6  "<fh>"
  DCDI/1 -> Mux1/1  "CD_f"
  Constant1/1 -> Mux1/2  "CY_f"
  DCL/1 -> Mux1/3  "CL_f"
  Bus Selector1/8 -> DCL/8  "<fd_f>"
  Bus Selector4/6 -> DCm/6  "<fh>"
  Bus Selector4/2 -> DCm/2  "<fa>"
  Bus Selector4/4 -> DCm/4  "<fm>"
  Bus Selector4/5 -> DCm/5  "<idxh>"
  Bus Selector4/8 -> DCm/8  "<fd_f>"
  Bus Selector4/1 -> DCm/1  "<idxa>"
  Bus Selector1/2 -> DCL/2  "<fa>"
  Bus Selector1/5 -> DCL/5  "<idxh>"
  Bus Selector1/1 -> DCL/1  "<idxa>"
  DCm/1 -> Mux1/5  "Cm_f"
  Mux1/1 -> delCoeff_f/1
  Bus Selector/6 -> DCDI/6  "<fh>"
  Bus Selector/8 -> DCDI/8  "<fd_f>"
  Bus Selector/1 -> DCDI/1  "<idxa>"
  Bus Selector/2 -> DCDI/2  "<fa>"
  Bus Selector/5 -> DCDI/5  "<idxh>"
  Bus Selector/4 -> DCDI/4  "<fm>"

== system AFDNFSmodelMPA/Nonlinear Flight Simulator/Forces&Moments/Digital DATCOM v1.0.2/Dynamic Contribution/Aerodynamic Forces and Moments Stability Axis/CG-CP Transformation ==
  Vb : Inport
  Property-In-Stability (PIS) : Inport  Port=2
  Body2Stability : Subsystem
  "Incidence, Sideslip, & Airspeed" : Subsystem
      mask Display:
      | port_label('input',1,'V_b','texmode','on');
      | port_label('output',1,'\alpha','texmode','on');
      | port_label('output',2,'\beta','texmode','on');
      | port_label('output',3,'V','texmode','on');
  Product : Product  Multiplication=Matrix(*)  RndMeth=Zero
  Terminator : Terminator
  Terminator1 : Terminator
  Transpose : Math  Operator=transpose  SaturateOnIntegerOverflow=on
  Property-In-Body (PIB) : Outport
  wires:
  Product/1 -> Property-In-Body (PIB)/1
  Property-In-Stability (PIS)/1 -> Product/2
  "Incidence, Sideslip, & Airspeed"/1(Alpha) -> Body2Stability/1(alpha)
  Body2Stability/1(Ts/b) -> Transpose/1
  Transpose/1 -> Product/1  "Stability2Body"
  Vb/1 -> "Incidence, Sideslip, & Airspeed"/1(Vb)
  "Incidence, Sideslip, & Airspeed"/2(Beta) -> Terminator/1
  "Incidence, Sideslip, & Airspeed"/3(V) -> Terminator1/1

== system AFDNFSmodelMPA/Nonlinear Flight Simulator/Forces&Moments/Digital DATCOM v1.0.2/Dynamic Contribution/Aerodynamic Forces and Moments Stability Axis/Force Transformation ==
  Vb : Inport
  Property-In-Stability (PIS) : Inport  Port=2
  Body2Stability : Subsystem
  "Incidence, Sideslip, & Airspeed" : Subsystem
      mask Display:
      | port_label('input',1,'V_b','texmode','on');
      | port_label('output',1,'\alpha','texmode','on');
      | port_label('output',2,'\beta','texmode','on');
      | port_label('output',3,'V','texmode','on');
  Product : Product  Multiplication=Matrix(*)  RndMeth=Zero
  Terminator : Terminator
  Terminator1 : Terminator
  Transpose : Math  Operator=transpose  SaturateOnIntegerOverflow=on
  Property-In-Body (PIB) : Outport
  wires:
  Product/1 -> Property-In-Body (PIB)/1
  Property-In-Stability (PIS)/1 -> Product/2
  "Incidence, Sideslip, & Airspeed"/1(Alpha) -> Body2Stability/1(alpha)
  Body2Stability/1(Ts/b) -> Transpose/1
  Transpose/1 -> Product/1  "Stability2Body"
  Vb/1 -> "Incidence, Sideslip, & Airspeed"/1(Vb)
  "Incidence, Sideslip, & Airspeed"/2(Beta) -> Terminator/1
  "Incidence, Sideslip, & Airspeed"/3(V) -> Terminator1/1

== system AFDNFSmodelMPA/Nonlinear Flight Simulator/Forces&Moments/Digital DATCOM v1.0.2/Dynamic Contribution/Aerodynamic Forces and Moments Stability Axis/Moment Transformation ==
  Vb : Inport
  Property-In-Stability (PIS) : Inport  Port=2
  Body2Stability : Subsystem
  "Incidence, Sideslip, & Airspeed" : Subsystem
      mask Display:
      | port_label('input',1,'V_b','texmode','on');
      | port_label('output',1,'\alpha','texmode','on');
      | port_label('output',2,'\beta','texmode','on');
      | port_label('output',3,'V','texmode','on');
  Product : Product  Multiplication=Matrix(*)  RndMeth=Zero
  Terminator : Terminator
  Terminator1 : Terminator
  Transpose : Math  Operator=transpose  SaturateOnIntegerOverflow=on
  Property-In-Body (PIB) : Outport
  wires:
  "Incidence, Sideslip, & Airspeed"/3(V) -> Terminator1/1
  "Incidence, Sideslip, & Airspeed"/2(Beta) -> Terminator/1
  Vb/1 -> "Incidence, Sideslip, & Airspeed"/1(Vb)
  Transpose/1 -> Product/1  "Stability2Body"
  Body2Stability/1(Ts/b) -> Transpose/1
  "Incidence, Sideslip, & Airspeed"/1(Alpha) -> Body2Stability/1(alpha)
  Property-In-Stability (PIS)/1 -> Product/2
  Product/1 -> Property-In-Body (PIB)/1

== system AFDNFSmodelMPA/Nonlinear Flight Simulator/Forces&Moments/Digital DATCOM v1.0.2/Static Contribution/Aerodynamic Forces and Moments/CG-CP Transformation ==
  Vb : Inport
  Property-In-Stability (PIS) : Inport  Port=2
  Body2Stability : Subsystem
  "Incidence, Sideslip, & Airspeed" : Subsystem
      mask Display:
      | port_label('input',1,'V_b','texmode','on');
      | port_label('output',1,'\alpha','texmode','on');
      | port_label('output',2,'\beta','texmode','on');
      | port_label('output',3,'V','texmode','on');
  Product : Product  Multiplication=Matrix(*)  RndMeth=Zero
  Terminator : Terminator
  Terminator1 : Terminator
  Transpose : Math  Operator=transpose  SaturateOnIntegerOverflow=on
  Property-In-Body (PIB) : Outport
  wires:
  Product/1 -> Property-In-Body (PIB)/1
  Property-In-Stability (PIS)/1 -> Product/2
  "Incidence, Sideslip, & Airspeed"/1(Alpha) -> Body2Stability/1(alpha)
  Body2Stability/1(Ts/b) -> Transpose/1
  Transpose/1 -> Product/1  "Stability2Body"
  Vb/1 -> "Incidence, Sideslip, & Airspeed"/1(Vb)
  "Incidence, Sideslip, & Airspeed"/2(Beta) -> Terminator/1
  "Incidence, Sideslip, & Airspeed"/3(V) -> Terminator1/1

== system AFDNFSmodelMPA/Nonlinear Flight Simulator/Forces&Moments/Digital DATCOM v1.0.2/Static Contribution/Aerodynamic Forces and Moments/Force Transformation ==
  Vb : Inport
  Property-In-Stability (PIS) : Inport  Port=2
  Body2Stability : Subsystem
  "Incidence, Sideslip, & Airspeed" : Subsystem
      mask Display:
      | port_label('input',1,'V_b','texmode','on');
      | port_label('output',1,'\alpha','texmode','on');
      | port_label('output',2,'\beta','texmode','on');
      | port_label('output',3,'V','texmode','on');
  Product : Product  Multiplication=Matrix(*)  RndMeth=Zero
  Terminator : Terminator
  Terminator1 : Terminator
  Transpose : Math  Operator=transpose  SaturateOnIntegerOverflow=on
  Property-In-Body (PIB) : Outport
  wires:
  Product/1 -> Property-In-Body (PIB)/1
  Property-In-Stability (PIS)/1 -> Product/2
  "Incidence, Sideslip, & Airspeed"/1(Alpha) -> Body2Stability/1(alpha)
  Body2Stability/1(Ts/b) -> Transpose/1
  Transpose/1 -> Product/1  "Stability2Body"
  Vb/1 -> "Incidence, Sideslip, & Airspeed"/1(Vb)
  "Incidence, Sideslip, & Airspeed"/2(Beta) -> Terminator/1
  "Incidence, Sideslip, & Airspeed"/3(V) -> Terminator1/1

== system AFDNFSmodelMPA/Nonlinear Flight Simulator/Forces&Moments/Digital DATCOM v1.0.2/Static Contribution/Aerodynamic Forces and Moments/Moment Transformation ==
  Vb : Inport
  Property-In-Stability (PIS) : Inport  Port=2
  Body2Stability : Subsystem
  "Incidence, Sideslip, & Airspeed" : Subsystem
      mask Display:
      | port_label('input',1,'V_b','texmode','on');
      | port_label('output',1,'\alpha','texmode','on');
      | port_label('output',2,'\beta','texmode','on');
      | port_label('output',3,'V','texmode','on');
  Product : Product  Multiplication=Matrix(*)  RndMeth=Zero
  Terminator : Terminator
  Terminator1 : Terminator
  Transpose : Math  Operator=transpose  SaturateOnIntegerOverflow=on
  Property-In-Body (PIB) : Outport
  wires:
  "Incidence, Sideslip, & Airspeed"/3(V) -> Terminator1/1
  "Incidence, Sideslip, & Airspeed"/2(Beta) -> Terminator/1
  Vb/1 -> "Incidence, Sideslip, & Airspeed"/1(Vb)
  Transpose/1 -> Product/1  "Stability2Body"
  Body2Stability/1(Ts/b) -> Transpose/1
  "Incidence, Sideslip, & Airspeed"/1(Alpha) -> Body2Stability/1(alpha)
  Property-In-Stability (PIS)/1 -> Product/2
  Product/1 -> Property-In-Body (PIB)/1
